simulink model "FM_Bistatic_Radar_Full"  (R2025a)
settings: Solver=VariableStepAuto  StartTime=0.0  StopTime=10.0  RelTol=1e-3
libraries: dspadpt3 x1, commanabbnd3 x1
(part 3 of 3)

== system FM_Bistatic_Radar_Full/Adaptive Filter/Gradiant Adaptive Lattice/50-Stage Lattice Predictor/Stage 5/K Update Equation ==
  F I/P : Inport
  B I/P : Inport  Port=2
  K I/P : Inport  Port=3
  Conjugate : Math  Operator=conj  SignedPower=on  RndMeth=Zero
  Conjugate1 : Math  Operator=conj  SignedPower=on  RndMeth=Zero
  Constant : Constant  Value=0.01
  Dot Product : DotProduct  OutDataTypeStr=Inherit: Inherit via internal rule
  Dot Product1 : DotProduct  OutDataTypeStr=Inherit: Inherit via internal rule
  Subtract : Sum  Inputs=+-
  *K (K conjugate) : Outport
  K : Outport  Port=2
  wires:
  F I/P/1 -> Dot Product/1
  B I/P/1 -> Conjugate/1
  Conjugate/1 -> Dot Product/2
  Constant/1 -> Dot Product1/2
  Dot Product/1 -> Dot Product1/1
  Conjugate1/1 -> *K (K conjugate)/1
  Dot Product1/1 -> Subtract/2
  Subtract/1 -> K/1, Conjugate1/1
  K I/P/1 -> Subtract/1

== system FM_Bistatic_Radar_Full/Adaptive Filter/Gradiant Adaptive Lattice/50-Stage Lattice Predictor/Stage 50/K Update Equation ==
  F I/P : Inport
  B I/P : Inport  Port=2
  K I/P : Inport  Port=3
  Conjugate : Math  Operator=conj  SignedPower=on  RndMeth=Zero
  Conjugate1 : Math  Operator=conj  SignedPower=on  RndMeth=Zero
  Constant : Constant  Value=0.01
  Dot Product : DotProduct  OutDataTypeStr=Inherit: Inherit via internal rule
  Dot Product1 : DotProduct  OutDataTypeStr=Inherit: Inherit via internal rule
  Subtract : Sum  Inputs=+-
  *K (K conjugate) : Outport
  K : Outport  Port=2
  wires:
  F I/P/1 -> Dot Product/1
  B I/P/1 -> Conjugate/1
  Conjugate/1 -> Dot Product/2
  Constant/1 -> Dot Product1/2
  Dot Product/1 -> Dot Product1/1
  Conjugate1/1 -> *K (K conjugate)/1
  Dot Product1/1 -> Subtract/2
  Subtract/1 -> K/1, Conjugate1/1
  K I/P/1 -> Subtract/1

== system FM_Bistatic_Radar_Full/Adaptive Filter/Gradiant Adaptive Lattice/50-Stage Lattice Predictor/Stage 51/K Update Equation ==
  F I/P : Inport
  B I/P : Inport  Port=2
  K I/P : Inport  Port=3
  Conjugate : Math  Operator=conj  SignedPower=on  RndMeth=Zero
  Conjugate1 : Math  Operator=conj  SignedPower=on  RndMeth=Zero
  Constant : Constant  Value=0.01
  Dot Product : DotProduct  OutDataTypeStr=Inherit: Inherit via internal rule
  Dot Product1 : DotProduct  OutDataTypeStr=Inherit: Inherit via internal rule
  Subtract : Sum  Inputs=+-
  *K (K conjugate) : Outport
  K : Outport  Port=2
  wires:
  F I/P/1 -> Dot Product/1
  B I/P/1 -> Conjugate/1
  Conjugate/1 -> Dot Product/2
  Constant/1 -> Dot Product1/2
  Dot Product/1 -> Dot Product1/1
  Conjugate1/1 -> *K (K conjugate)/1
  Dot Product1/1 -> Subtract/2
  Subtract/1 -> K/1, Conjugate1/1
  K I/P/1 -> Subtract/1

== system FM_Bistatic_Radar_Full/Adaptive Filter/Gradiant Adaptive Lattice/50-Stage Lattice Predictor/Stage 6/K Update Equation ==
  F I/P : Inport
  B I/P : Inport  Port=2
  K I/P : Inport  Port=3
  Conjugate : Math  Operator=conj  SignedPower=on  RndMeth=Zero
  Conjugate1 : Math  Operator=conj  SignedPower=on  RndMeth=Zero
  Constant : Constant  Value=0.01
  Dot Product : DotProduct  OutDataTypeStr=Inherit: Inherit via internal rule
  Dot Product1 : DotProduct  OutDataTypeStr=Inherit: Inherit via internal rule
  Subtract : Sum  Inputs=+-
  *K (K conjugate) : Outport
  K : Outport  Port=2
  wires:
  F I/P/1 -> Dot Product/1
  B I/P/1 -> Conjugate/1
  Conjugate/1 -> Dot Product/2
  Constant/1 -> Dot Product1/2
  Dot Product/1 -> Dot Product1/1
  Conjugate1/1 -> *K (K conjugate)/1
  Dot Product1/1 -> Subtract/2
  Subtract/1 -> K/1, Conjugate1/1
  K I/P/1 -> Subtract/1

== system FM_Bistatic_Radar_Full/Adaptive Filter/Gradiant Adaptive Lattice/50-Stage Lattice Predictor/Stage 7/K Update Equation ==
  F I/P : Inport
  B I/P : Inport  Port=2
  K I/P : Inport  Port=3
  Conjugate : Math  Operator=conj  SignedPower=on  RndMeth=Zero
  Conjugate1 : Math  Operator=conj  SignedPower=on  RndMeth=Zero
  Constant : Constant  Value=0.01
  Dot Product : DotProduct  OutDataTypeStr=Inherit: Inherit via internal rule
  Dot Product1 : DotProduct  OutDataTypeStr=Inherit: Inherit via internal rule
  Subtract : Sum  Inputs=+-
  *K (K conjugate) : Outport
  K : Outport  Port=2
  wires:
  F I/P/1 -> Dot Product/1
  B I/P/1 -> Conjugate/1
  Conjugate/1 -> Dot Product/2
  Constant/1 -> Dot Product1/2
  Dot Product/1 -> Dot Product1/1
  Conjugate1/1 -> *K (K conjugate)/1
  Dot Product1/1 -> Subtract/2
  Subtract/1 -> K/1, Conjugate1/1
  K I/P/1 -> Subtract/1

== system FM_Bistatic_Radar_Full/Adaptive Filter/Gradiant Adaptive Lattice/50-Stage Lattice Predictor/Stage 8/K Update Equation ==
  F I/P : Inport
  B I/P : Inport  Port=2
  K I/P : Inport  Port=3
  Conjugate : Math  Operator=conj  SignedPower=on  RndMeth=Zero
  Conjugate1 : Math  Operator=conj  SignedPower=on  RndMeth=Zero
  Constant : Constant  Value=0.01
  Dot Product : DotProduct  OutDataTypeStr=Inherit: Inherit via internal rule
  Dot Product1 : DotProduct  OutDataTypeStr=Inherit: Inherit via internal rule
  Subtract : Sum  Inputs=+-
  *K (K conjugate) : Outport
  K : Outport  Port=2
  wires:
  F I/P/1 -> Dot Product/1
  B I/P/1 -> Conjugate/1
  Conjugate/1 -> Dot Product/2
  Constant/1 -> Dot Product1/2
  Dot Product/1 -> Dot Product1/1
  Conjugate1/1 -> *K (K conjugate)/1
  Dot Product1/1 -> Subtract/2
  Subtract/1 -> K/1, Conjugate1/1
  K I/P/1 -> Subtract/1

== system FM_Bistatic_Radar_Full/Adaptive Filter/Gradiant Adaptive Lattice/50-Stage Lattice Predictor/Stage 9/K Update Equation ==
  F I/P : Inport
  B I/P : Inport  Port=2
  K I/P : Inport  Port=3
  Conjugate : Math  Operator=conj  SignedPower=on  RndMeth=Zero
  Conjugate1 : Math  Operator=conj  SignedPower=on  RndMeth=Zero
  Constant : Constant  Value=0.01
  Dot Product : DotProduct  OutDataTypeStr=Inherit: Inherit via internal rule
  Dot Product1 : DotProduct  OutDataTypeStr=Inherit: Inherit via internal rule
  Subtract : Sum  Inputs=+-
  *K (K conjugate) : Outport
  K : Outport  Port=2
  wires:
  F I/P/1 -> Dot Product/1
  B I/P/1 -> Conjugate/1
  Conjugate/1 -> Dot Product/2
  Constant/1 -> Dot Product1/2
  Dot Product/1 -> Dot Product1/1
  Conjugate1/1 -> *K (K conjugate)/1
  Dot Product1/1 -> Subtract/2
  Subtract/1 -> K/1, Conjugate1/1
  K I/P/1 -> Subtract/1

== matlab function FM_Bistatic_Radar_Full/Source & Channel & Backscatter/MATLAB Function ==
  data: u input; y output
function y = fcn(u)
    
y = u;

== matlab function FM_Bistatic_Radar_Full/Source & Channel & Backscatter/MATLAB Function1 ==
  data: u input; y output
function y = fcn(u)

y = u;
